simulink model "sensorFusionWithControlTB66State"  (R2024a)
settings: Solver=FixedStepAuto  StartTime=0.0  StopTime=inf  FixedStep=controlRate  RelTol=1e-3
InitFcn:
  | modelParamsDD = Simulink.data.dictionary.open('modelConfigData.sldd');
  | sectModel = getSection(modelParamsDD,'Design Data');
  | controlRateTemp = getValue(getEntry(sectModel,'controlRate'));
  | mpcRate = getValue(getEntry(sectModel,'mpcRate'));
  | 
  | measRate = controlRateTemp;
  | angleEstRate = measRate;
  | stateEstRate = measRate;
  | 
  | % Complementary filter
  | fc = 5; %Hz
  | tau = 1/(2*pi*fc);
  | % alpha = tau/(tau+controlRateTemp);
  | alpha = 0.98;
  | 
  | % Control params
  | tiltSetPoint = 5; % degree
  | 
  | % Motor params
  | % PPR = 13;
  | % gearReductionRatio = 42;
  | % ABPhase = 4;
  | 
  | % Tilt angle PID
  | Tw = 1;
  | Kp = 25;
  | Ki = 15; % At 100 Hz
  | Kd = 0;
  | 
  | clear controlRateTemp
  | 
  | motorParamsDD = Simulink.data.dictionary.open('motorParametersData.sldd');
  | robotParamsDD = Simulink.data.dictionary.open('robotModelData.sldd');
  | % controlParamsDD = Simulink.data.dictionary.open('controlVariablesData.sldd');
  | sectMotor = getSection(motorParamsDD,'Design Data');
  | sectRobot = getSection(robotParamsDD,'Design Data');
  | % sectControl = getSection(controlParamsDD,'Design Data');
  | 
  | % Physical Parameters
  | M = getValue(getEntry(sectRobot,'massOfCart'));    % mass of cart
  | m = getValue(getEntry(sectRobot,'massOfPendulum'));    % mass of pendulum
  | L = getValue(getEntry(sectRobot,'lengthToPendulumCenterOfMass'));    % length to pendulum center of mass
  | g = 9.81;   % gravity
  | I = getValue(getEntry(sectRobot,'inertiaOfPendulum'));  % inertia of pendulum
  | r = getValue(getEntry(sectRobot,'wheelRadius'));   % 5 cm wheel radius
  | 
  | % Servo motor state: i, omega
  | Rm = getValue(getEntry(sectMotor,'armatureResistance')); % motor resistance
  | Lm = getValue(getEntry(sectMotor,'armatureInductance')); % motor coil inductance
  | Km = getValue(getEntry(sectMotor,'motorTorqueConstantKm')); % motor torque constant
  | Kb = getValue(getEntry(sectMotor,'backEMFConstantKb')); % motor electrical consant
  | Kf = getValue(getEntry(sectMotor,'viscousFriction')); % viscous friction
  | J = getValue(getEntry(sectMotor,'motorInertia'));  % inertia of rotor
  | 
  | % Q_aug_lqr_temp = getValue(getEntry(sectControl,'Q_aug_lqr'));
  | % R_aug_lqr_temp = getValue(getEntry(sectControl,'R_aug_lqr'));
  | 
  | % States are x, dx/dt, phi, dphi/dt
  | % Outputs are x position and tilt angle
  | 
  | % Linearized state-space model of inverted pendulum
  | I_tot = m*L^2+I;
  | p = m^2*L^2 - I_tot*(M+m);
  | A_pend = [0 1 0 0;
  |           0 0 (m^2 * g * L^2)/p 0;
  |           0 0 0 1;
  |           0 0 -(M+m)/(m*L)*m^2*L^2*g/p 0];
  | 
  | B_pend = [0; -I_tot/p; 0; 1/(m*L)*(1+(M+m)*I_tot/p)];
  | 
  | C_pend = [1 0 0 0;
  |           0 0 1 0];
  | D_pend = zeros(2,1);
  | 
  | % Discretize System - for the augmented system
  | sysd = c2d(ss(A_pend, B_pend, C_pend, D_pend), measRate);
  | Ad_pend = single(sysd.A);
  | Bd_pend = single(sysd.B);
  | Cd_pend = single(sysd.C);
  | Dd_pend = single(sysd.D);
  | 
  | % State-space model: output is torque = Km * i
  | A_motor = [-Rm/L,   -Kb/Lm;
  |             Km/J, -Kf/J];
  | B_motor = [1/Lm;
  |            0];
  | C_motor = [Km*(1/r), 0];  % Output is torque = Km * i
  | D_motor = 0;
  | 
  | % Augment System: Force = torque / r
  | % States are x, dx/dt, phi, dphi/dt, i, w
  | % Outputs are x position and tilt angle
  | 
  | A_aug = [A_pend, B_pend*C_motor;
  |          zeros(2,4), A_motor];
  | 
  | B_aug = [B_pend*D_motor; B_motor];
  | 
  | C_aug = [C_pend, D_pend*C_motor];
  | n_aug = size(A_aug,1);
  | 
  | 
  | % Discretize System - for the augmented system
  | sysd = c2d(ss(A_aug, B_aug, C_aug, 0), measRate);
  | Ad_aug = single(sysd.A);
  | Bd_aug = single(sysd.B);
  | Cd_aug = single(sysd.C);
  | 
  | clear J Kt M m l g I r Q_lqr_temp R_lqr_temp dt
  | clear Rm Lm Km Kb Kf J
  | clear motorParamsDD robotParamsDD controlParamsDD modelParamsDD sectMotor sectRobot sectControl sectModel sysd
  | 
  | % LQR Controller matrices (moved here from SLDD to be tuned)
  | xm = 0.01;
  | xdm = 2;
  | pm = 0.2;
  | pdm = 5;
  | im = 2;
  | wm = 100;
  | 
  | Q_aug_lqr_temp = 0.1*diag([(1/xm)^2,(1/xdm)^2,(1/pm)^2,(1/pdm)^2,(1/im)^2,(1/wm)^2]);
  | R_aug_lqr_temp = 15;
  | 
  | % LQR Controller - for the augmented system
  | [K_aug_lqr, ~, ~] = dlqr(Ad_aug, Bd_aug, Q_aug_lqr_temp, R_aug_lqr_temp);
  | K_aug_lqr = single(K_aug_lqr);
  | 
  | clear Q_aug_lqr_temp R_aug_lqr_temp
  | 
  | %% MPC Tuning:
  | % Control Voltage was low, settling of the state variables is slow.
  | % Sol1: Decrease mpc1.Weights.MVRate (the penalty on voltage be cheaper)
  | % Sol2: Increase the weights penalty (same, more expensive error)
  | % Sol3: Initial conditions should not be near the constraints.
  | 
  | % For 1000 Hz sample rate with sensors, and 100 Hz sample rate MPC, the
  | % 200 long predict and 10 long control horizon should be enough,
  | % the system can't change faster.
  | 
  | % MPC tuning params
  | horizonNum = 100;
  | controlHorizon = 20;
  | 
  | MVWeight = 0;
  | MVRateWeight = 0.1;
  | stateVariableWeights = [0 0 1 0 0 0];
  | ECR = 100000;
  | 
  | % MPC Constraints
  | x_m = 2;
  | x_dot_m = 2;
  | phi_m = 1;
  | phi_dot_m = 35;
  | i_m = 10;
  | w_m = 200;
  | 
  | % MPC
  | robSys_mpc = c2d(ss(A_aug, B_aug, eye(6), zeros(6,1)), mpcRate);
  | %% create MPC controller object with sample time
  | mpc1 = mpc(robSys_mpc, mpcRate);
  | %% specify prediction horizon
  | mpc1.PredictionHorizon = horizonNum;
  | %% specify control horizon
  | mpc1.ControlHorizon = controlHorizon;
  | %% specify nominal values for inputs and outputs
  | mpc1.Model.Nominal.U = 0;
  | mpc1.Model.Nominal.Y = [0;0;0;0;0;0];
  | %% specify constraints for MV and MV Rate
  | mpc1.MV(1).Min = -12;
  | mpc1.MV(1).Max = 12;
  | %% specify constraints for OV
  | mpc1.OV(1).Min = -x_m;
  | mpc1.OV(1).Max = x_m;
  | mpc1.OV(2).Min = -x_dot_m;
  | mpc1.OV(2).Max = x_dot_m;
  | mpc1.OV(3).Min = -phi_m;
  | mpc1.OV(3).Max = phi_m;
  | mpc1.OV(4).Min = -phi_dot_m;
  | mpc1.OV(4).Max = phi_dot_m;
  | mpc1.OV(5).Min = -i_m;
  | mpc1.OV(5).Max = i_m;
  | mpc1.OV(6).Min = -w_m;
  | mpc1.OV(6).Max = w_m;
  | %% specify weights
  | mpc1.Weights.MV = MVWeight;
  | mpc1.Weights.MVRate = MVRateWeight;
  | mpc1.Weights.OV = stateVariableWeights;
  | mpc1.Weights.ECR = ECR;
  | %% specify overall adjustment factor applied to estimation model gains
  | alphaMPC = 4.1687;
  | %% adjust default output disturbance model gains
  | setoutdist(mpc1, 'model', getoutdist(mpc1)*0);
  | %% adjust default measurement noise model gains
  | mpc1.Model.Noise = mpc1.Model.Noise*0;
  | %% specify simulation options
  | options = mpcsimopt();
  | options.RefLookAhead = 'off';
  | options.MDLookAhead = 'off';
  | options.Constraints = 'on';
  | options.OpenLoop = 'off';
  | 
  | setEstimator(mpc1,'custom')
undefined symbols (not defined in the file or in its folder): accelToUnit, controlRate, gyroToUnit, MaxMotorVoltage
libraries: stm32blockslib x2, stm32f7xxblockslib x2, stm32f4xxblockslib x1
settings Model: DataDictionary=globalData.sldd  VariantConfigurationObject=RobotVariantConfig  STM32="{\"PWMOutput\":[{\"ID\":\"sensorFusionWithControlTB66State:205\"},{\"ID\":\"sensorFusionWithControlTB66State:189\"}],\"DigitalPortWrite\":[{\"ID\":\"sensorFusionWithControlTB66State:1189\"},{\"ID\":\"sensorFusionWithControlTB66State:1225:7\"},{\"ID\":\"sensorFusionWithControlTB66State:1225:8\"},{\"ID\":\"sensorFusionWithControlTB66State:1225:9\"},{\"ID\":\"sensorFusionWithControlTB66State:1225:10\"}],\"EncoderBlock\":[{\"ID\":\"sensorFusionWithControlTB66State:1254\"},{\"ID\":\"sensorFusionWithControlTB66State:1257\"}],\"I2CControllerRead\":[{\"ID\":\"sensorFusionWithControlTB66State:1237:7\"},{\"ID\":\"sensorFusionWithControlTB66State:1237:18\"},{\"ID\":\"sensorFusionWithControlTB66State:1237:19\"},{\"ID\":\"sensorFusionWithControlTB66State:1237:20\"},{\"ID\":\"sensorFusionWithControlTB66State:1238:7\"},{\"ID\":\"sensorFusionWithControlTB66State:1238:15\"},{\"ID\":\"sensorFusionWithControlTB66State:1238:16\"},{\"ID\":\"sensorFusionWithControlTB66State:1238:17\"}],\"I2CControllerWrite\":[{\"ID\":\"sensorFusionWithControlTB66State:1237:21\"},{\"ID\":\"sensorFusionWithControlTB66State:1237:22\"},{\"ID\":\"sensorFusionWithControlTB66State:1237:23\"},{\"ID\":\"sensorFusionWithControlTB66State:1238:18\"},{\"ID\":\"sensorFusionWithControlTB66State:1238:19\"},{\"ID\":\"sensorFusionWithControlTB66State:1238:20\"}]}"  SimulationMode=external  Creator=Peter  LastModifiedBy=Peter
settings SolverCC: PositivePriorityOrder=on
settings OptimizationCC: OptimizeBlockIOStorage=off  BufferReuse=off  ReuseModelBlockBuffer=off  GlobalBufferReuse=off  ExpressionFolding=off  EnableMemcpy=off  PassReuseOutputArgsAs=Individual arguments  LocalBlockOutputs=off  ZeroExternalMemoryAtStartup=off  ZeroInternalMemoryAtStartup=off  MaxStackSize=64  OptimizeDataStoreBuffers=off  BusAssignmentInplaceUpdate=off  OptimizationLevel=level0  OptimizationCustomize=off  EfficientTunableParamExpr=on
settings DebuggingCC: ParameterTunabilityLossMsg=error
settings HardwareCC: ProdBitPerPointer=32  ProdBitPerSizeT=32  ProdBitPerPtrDiffT=32  ProdLargestAtomicInteger=Long  ProdLargestAtomicFloat=Double  ProdWordSize=32  ProdLongLongMode=on  ProdHWDeviceType=ARM Compatible->ARM Cortex-M
settings SFSimCC: MATLABDynamicMemAlloc=off
settings RTWCC: Description=Embedded Coder  SystemTargetFile=ert.tlc  HardwareBoard=STM32F7xx Based (Single precision FPU)  TemplateMakefile=ert_default_tmf  Toolchain=GNU Tools for ARM Embedded Processors
settings CodeAppCC: GenerateComments=off  IgnoreCustomStorageClasses=off  OperatorAnnotations=on  SimulinkDataObjDesc=on  SFDataObjDesc=on  SimulinkBlockComments=off
settings ERTTargetCC: TargetLangStandard=C99 (ISO)  CodeReplacementLibrary=ARM Cortex-M  SupportComplex=off  ExtMode=on  ExtModeTransport=3  ExtModeStaticAlloc=on  ExtModeStaticAllocSize=2048  ExtModeMexFile=ext_xcp  ExtModeMexArgs=1 'COM11' 115200  ExtModeIntrfLevel=Level2 - Open

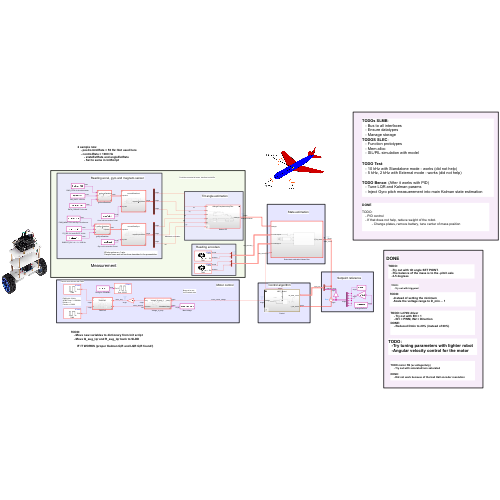
[thumbnail: Simulink's stored preview of the top-level diagram]
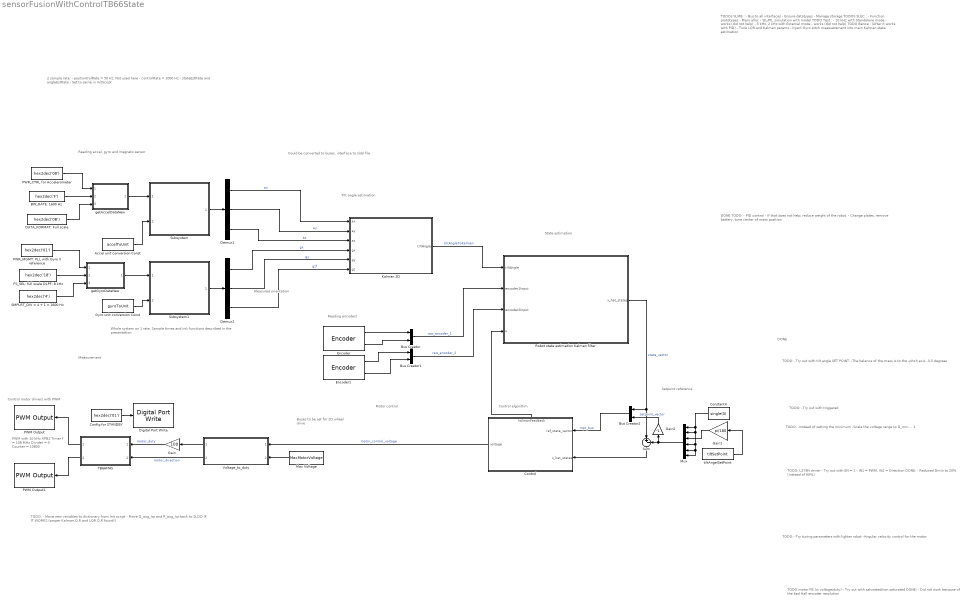
== system sensorFusionWithControlTB66State ==
  note: 2 sample rate:
      | - posControlRate = 50 Hz: Not used here
      | - controlRate = 1000 Hz
      | - stateEstRate and angleEstRate
      | - Set to same in InitScript
  note: Measured orientation
  note: PWM with 10 kHz
      | APB2 Timer f = 108 MHz
      | Divider = 0
      | Counter = 10800
  note: Measurement
  note: Motor control
  note: Tilt angle estimation
  note: Control motor dirvers with PWM
  note: Reading accel, gyro and megneto sensor
  note: Control algorithm
  note: Reading encoders
  note: State estimation
  note: Setpoint reference
  note: Could be converted to buses, interface to sldd file
  note: Whole system on 1 rate.
      | Sample times and init functions described in the presentation.
  note: Buses to be set
      | for 2D wheel drive
  note: TODO:
      | -Try tuning parameters with lighter robot
      | -Angular velocity control for the motor
  note: TODO motor FB (w voltage/duty)
      | - Try out with saturated/non saturated
      |
      | DONE:
      | - Did not work because of the bad Hall encoder resolution
  note: TODO:
      | -Try out with tilt angle SET POINT.
      | -The balance of the mass is to the -pitch axis
      | -3-5 degrees
  note: TODO: L279N driver
      | - Try out with EN = 1
      | - IN1 = PWM, IN2 = Direction
      | DONE:
      | - Reduced Dmin to 20% (instead of 60%)
  note: TODOs SLMB :
      | - Bus to all interfaces
      | - Ensure datatypes
      | - Manage storage
      | TODOS SLEC :
      | - Function prototypes
      | - Mem alloc
      | - SIL/PIL simulation with model
      |
      | TODO Test :
      | - 10 kHz with Standalone mode - works (did not help)
      | - 5 kHz, 2 kHz with External mode - works (did not help)
      |
      | TODO Bence : (After it works with PID)
      | - Tune LQR and Kalman params
      | - Inject Gyro pitch measuerement into main Kalman state estimation
  note: TODO:
      | -Try out with triggered
  note: DONE
  note: DONE
      |
      | TODO:
      | - PID control
      | - If that does not help, reduce weight of the robot.
      | - Change plates, remove battery, tune center of mass position
  note: TODO:
      | -Instead of setting the minimum
      | -Scale the voltage range to D_min ... 1
  note: TODO:
      | - Move new variables to dictionary from Init script
      | - Move Q_aug_lqr and R_aug_lqr back to SLDD
      |
      | IF IT WORKS (proper Kalman Q,R and LQR Q,R found!)
  Accel unit conversion Const : Constant  Value=accelToUnit  OutDataTypeStr=single
  BW_RATE: 1600 Hz : Constant  Value=hex2dec('F')  OutDataTypeStr=uint8
  Bus Creator : BusCreator  Inputs=2
  Bus Creator1 : BusCreator  Inputs=2
  Bus Creator2 : BusCreator  Inputs=2
  Config for STANDBY : Constant  Value=hex2dec('01')  OutDataTypeStr=uint8
  Constant4 : Constant  Value=single(0)
  Control : Subsystem  Variant=on  VariantChoicesEnumeration=controlEnumState  VariantControlVariable=controlAlgStateCtrl  VariantControl=Subsystem2  VariantActivationTime=inherit from Simulink.VariantControl
      settings: PortSchema="{\"entries\":[{\"content\":{\"sides\":[{\"content\":{\"connectorIds\":[\"In1\",\"In2\"]},\"type\":\"ConnectorPlacement.EquallySpacedRectSide\",\"uuid\":\"f699f757-4844-4aff-9ceb-41d5b2044f89\"},{\"content\":{\"connectorIds\":[\"Out1\"],\"side\":\"RIGHT\"},\"type\":\"ConnectorPlacement.EquallySpacedRectSide\",\"uuid\":\"5d4ff76b-5e14-4a3a-b7d6-9f05c394657c\"},{\"content\":{\"connectorIds\":[\"Out2\"],\"side\":\"TOP\"},\"type\":\"ConnectorPlacement.EquallySpacedRectSide\",\"uuid\":\"774b8687-b42a-4b88-b210-7c8eb4b61568\"}]},\"type\":\"ConnectorPlacement.EquallySpacedConnector\",\"uuid\":\"f6913896-c1bf-44b7-bb24-894f4bed7d15\"}],\"packageUris\":[\"http://schema.mathworks.com/mf0/Connector/R2020b\"],\"version\":\"1.0\"}"
  DATA_FORMAT: Full scale : Constant  Value=hex2dec('0B')  OutDataTypeStr=uint8
  Demux1 : Demux  Outputs=3
  Demux2 : Demux  Outputs=3
  Digital Port Write : stm32f4xxblockslib/Digital Port Write  PortName=GPIOF  PinNumber=[13]  ReadOperation=off  IOAsArray=off  EnableSimPort=off  hoistedMaskSrc=ECSoC/ECSimCodegen/Digital Port Write
      settings: LibrarySourceBlock=stm32f7xxblockslib/Digital Port Write
  Encoder : stm32blockslib/Encoder  TimerModule=TIM1  EnableResetInput=off  OutputDirection=on  SampleTime=angleEstRate
      settings: LibrarySourceBlock=stm32f7xxblockslib/Encoder
  Encoder1 : stm32blockslib/Encoder  TimerModule=TIM3  EnableResetInput=off  OutputDirection=on  SampleTime=angleEstRate
      settings: LibrarySourceBlock=stm32f7xxblockslib/Encoder
  FS_SEL: full scale DLPF: 8 kHz : Constant  Value=hex2dec('18')  OutDataTypeStr=uint8
  Gain : Gain  Gain=100
  Gain1 : Gain  Gain=pi/180  ParamDataTypeStr=single
  Gain2 : Gain  Gain=-1
  Gyro unit conversion Const : Constant  Value=gyroToUnit  OutDataTypeStr=single
  Kalman 2D : Subsystem  Variant=on  VariantChoicesEnumeration=tiltEnum  VariantControlVariable=tiltEstCtrl  VariantControl=Kalman 2D  VariantActivationTime=inherit from Simulink.VariantControl
  Max Voltage : Constant  Value=MaxMotorVoltage  OutDataTypeStr=single
  Mux : Mux  Inputs=6
  PWM Output : stm32f7xxblockslib/PWM Output  TimerModule=TIM8  DutycycleUnits=Percentage  EnableChannel1=off  EnableChannel2=off  EnableChannel3=on  EnableChannel4=off  EnableChannel5=off  EnableChannel6=off  EnableCounterInput=off  EnableMainOutputInput=off  EnableFrequencyInput=off  SetRCAfterCE=off  OutputDirection=off  OutputMainOutputEnableStatus=off  SampleTime=0.1  EnableSimPort=off  EnableUpdateEvent=off  EnableCaptureCompare1Event=off  EnableCaptureCompare2Event=off  EnableCaptureCompare3Event=off  EnableCaptureCompare4Event=off  EnableTriggerEvent=off  EnableBreakEvent=off  EnableBreakEvent2=off  ProcessorFamily=STM32F7  hoistedMaskSrc=ECSoC/ECSimCodegen/PWM Output
  PWM Output1 : stm32f7xxblockslib/PWM Output  TimerModule=TIM8  DutycycleUnits=Percentage  EnableChannel1=off  EnableChannel2=off  EnableChannel3=off  EnableChannel4=on  EnableChannel5=off  EnableChannel6=off  EnableCounterInput=off  EnableMainOutputInput=off  EnableFrequencyInput=off  SetRCAfterCE=off  OutputDirection=off  OutputMainOutputEnableStatus=off  SampleTime=0.1  EnableSimPort=off  EnableUpdateEvent=off  EnableCaptureCompare1Event=off  EnableCaptureCompare2Event=off  EnableCaptureCompare3Event=off  EnableCaptureCompare4Event=off  EnableTriggerEvent=off  EnableBreakEvent=off  EnableBreakEvent2=off  ProcessorFamily=STM32F7  hoistedMaskSrc=ECSoC/ECSimCodegen/PWM Output
  PWR_CTRL for Accelerometer : Constant  Value=hex2dec('08')  OutDataTypeStr=uint8
  PWR_MGMT: PLL with Gyro X reference : Constant  Value=hex2dec('01')  OutDataTypeStr=uint8
  Robot state estimation Kalman filter : Subsystem  TreatAsAtomicUnit=on  SystemSampleTime=stateEstRate
  SMPLRT_DIV = 4 + 1 = 1600 Hz : Constant  Value=hex2dec('4')  OutDataTypeStr=uint8
  Subsystem : Subsystem  TreatAsAtomicUnit=on  SystemSampleTime=angleEstRate  ReferencedSubsystem=convertRawAccel
  Subsystem1 : Subsystem  TreatAsAtomicUnit=on  SystemSampleTime=angleEstRate  ReferencedSubsystem=convertRawGyro
  Sum : Sum  Inputs=|+-
  TB66FNG : Subsystem  TreatAsAtomicUnit=on  SystemSampleTime=controlRate  ReferencedSubsystem=TB66FNG
  Voltage_to_duty : Subsystem  TreatAsAtomicUnit=on  SystemSampleTime=controlRate  ReferencedSubsystem=Voltage_to_duty_1
  getAccelDataNew : Subsystem  TreatAsAtomicUnit=on  ReferencedSubsystem=getAccelDataNew
  getGyroDataNew : Subsystem  TreatAsAtomicUnit=on  ReferencedSubsystem=getGyroDataNew
  tiltAngelSetPoint : Constant  Value=tiltSetPoint  OutDataTypeStr=single
  wires:
  Max Voltage/1 -> Voltage_to_duty/2
  Gyro unit conversion Const/1 -> Subsystem1/2
  Subsystem1/1 -> Demux2/1
  PWR_MGMT: PLL with Gyro X reference/1 -> getGyroDataNew/1
  getGyroDataNew/1 -> Subsystem1/1
  Kalman 2D/1(tiltAngle) -> Robot state estimation Kalman filter/1(tiltAngle)  "tiltAngleToKalman"
  Demux1/1 -> Kalman 2D/1(ax)  "ax"
  Demux1/2 -> Kalman 2D/2(ay)  "ay"
  Demux1/3 -> Kalman 2D/3(az)  "az"
  Demux2/3 -> Kalman 2D/6(gz)  "gzf"
  getAccelDataNew/1 -> Subsystem/1
  Accel unit conversion Const/1 -> Subsystem/2
  Subsystem/1 -> Demux1/1
  Control/1(voltage) -> Voltage_to_duty/1  "motor_control_voltage"
  Demux2/1 -> Kalman 2D/4(gx)  "gx"
  Demux2/2 -> Kalman 2D/5(gy)  "gy"
  BW_RATE: 1600 Hz/1 -> getAccelDataNew/2
  PWR_CTRL for Accelerometer/1 -> getAccelDataNew/1
  FS_SEL: full scale DLPF: 8 kHz/1 -> getGyroDataNew/2
  SMPLRT_DIV = 4 + 1 = 1600 Hz/1 -> getGyroDataNew/3
  Sum/1 -> Control/2(x_hat_states)
  Mux/1 -> Gain2/1, Sum/2
  Constant4/1 -> Mux/6, Mux/5, Mux/4, Mux/2, Mux/1
  tiltAngelSetPoint/1 -> Gain1/1
  Voltage_to_duty/1 -> Gain/1
  Voltage_to_duty/2 -> TB66FNG/2  "motor_direction"
  TB66FNG/1 -> PWM Output/1
  TB66FNG/2 -> PWM Output1/1
  Config for STANDBY/1 -> Digital Port Write/1
  DATA_FORMAT: Full scale/1 -> getAccelDataNew/3
  Gain1/1 -> Mux/3
  Encoder/1 -> Bus Creator/1
  Encoder1/1 -> Bus Creator1/1
  Bus Creator/1 -> Robot state estimation Kalman filter/2(encoder1Input)  "raw_encoder_1"
  Encoder/2 -> Bus Creator/2
  Encoder1/2 -> Bus Creator1/2
  Bus Creator1/1 -> Robot state estimation Kalman filter/3(encoder2Input)  "raw_encoder_2"
  Robot state estimation Kalman filter/1(x_hat_states) -> Sum/1, Bus Creator2/1  "state_vector"
  Gain/1 -> TB66FNG/1  "motor_duty"
  Bus Creator2/1 -> Control/1(ref_state_vector)  "mpc_bus"
  Control/2(kalmanFeedback) -> Robot state estimation Kalman filter/4(u)
  Gain2/1 -> Bus Creator2/2  "setpoint_vector"

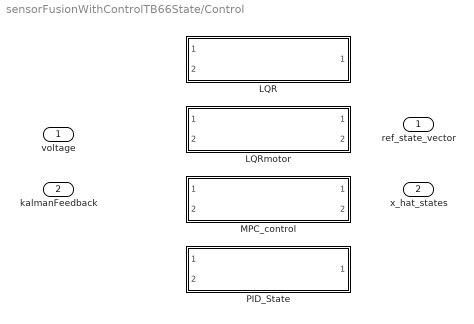
== system sensorFusionWithControlTB66State/Control ==
  ref_state_vector : Inport
  x_hat_states : Inport  Port=2  OutDataTypeStr=single
  LQR : Subsystem  SystemSampleTime=controlRate  VariantControl=controlAlgStateCtrl == controlEnumState.LQR  ReferencedSubsystem=LQR
  LQRmotor : Subsystem  SystemSampleTime=controlRate  VariantControl=controlAlgStateCtrl == controlEnumState.LQRmotor  ReferencedSubsystem=LQRmotor
  MPC_control : Subsystem  VariantControl=controlAlgStateCtrl == controlEnumState.MPC_control  ReferencedSubsystem=MPC_control
  PID_State : Subsystem  VariantControl=controlAlgStateCtrl == controlEnumState.PID_State  ReferencedSubsystem=PID_State
  voltage : Outport  OutDataTypeStr=single
  kalmanFeedback : Outport  Port=2  OutDataTypeStr=single

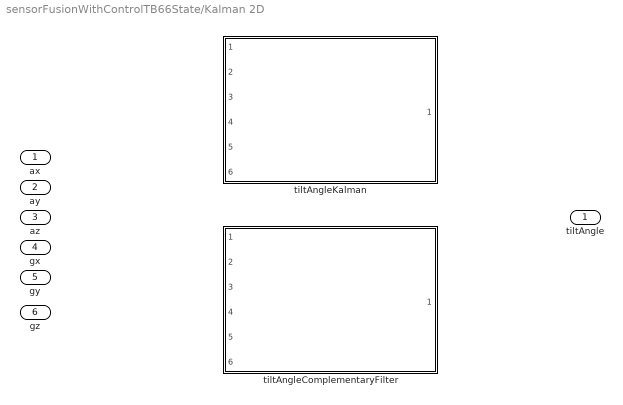
== system sensorFusionWithControlTB66State/Kalman 2D ==
  ax : Inport
  ay : Inport  Port=2
  az : Inport  Port=3
  gx : Inport  Port=4
  gy : Inport  Port=5
  gz : Inport  Port=6
  tiltAngleComplementaryFilter : Subsystem  TreatAsAtomicUnit=on  SystemSampleTime=controlRate  VariantControl=tiltEstCtrl == tiltEnum.tiltAngleComplementaryFilter  ReferencedSubsystem=tiltAngleComplementaryFilter
  tiltAngleKalman : Subsystem  TreatAsAtomicUnit=on  SystemSampleTime=angleEstRate  VariantControl=tiltEstCtrl == tiltEnum.tiltAngleKalman  ReferencedSubsystem=tiltAngleKalman
  tiltAngle : Outport

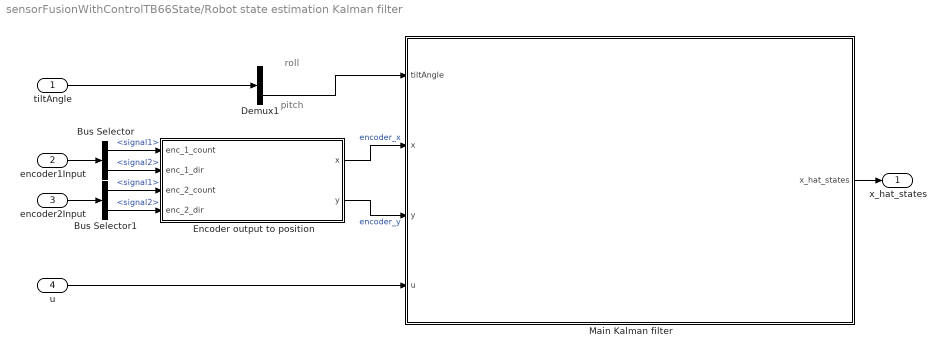
== system sensorFusionWithControlTB66State/Robot state estimation Kalman filter ==
  note: pitch
  note: roll
  tiltAngle : Inport
  encoder1Input : Inport  Port=2
  encoder2Input : Inport  Port=3
  u : Inport  Port=4
  Bus Selector : BusSelector  OutputSignals=signal1,signal2
  Bus Selector1 : BusSelector  OutputSignals=signal1,signal2
  Demux1 : Demux  Outputs=2
  Encoder output to position : Subsystem  Variant=on  VariantChoicesEnumeration=encoderDimEnum  VariantControlVariable=encoderDimCtrl  VariantControl=Encoder output to position  VariantActivationTime=inherit from Simulink.VariantControl
  Main Kalman filter : Subsystem  Variant=on  VariantChoicesEnumeration=mainStateEnum  VariantControlVariable=mainStateEstCtrl  VariantControl=Subsystem1  VariantActivationTime=inherit from Simulink.VariantControl
  x_hat_states : Outport  OutDataTypeStr=single
  wires:
  tiltAngle/1 -> Demux1/1
  Main Kalman filter/1(x_hat_states) -> x_hat_states/1
  Bus Selector/1 -> Encoder output to position/1(enc_1_count)  "<signal1>"
  Bus Selector/2 -> Encoder output to position/2(enc_1_dir)  "<signal2>"
  Encoder output to position/1(x) -> Main Kalman filter/2(x)  "encoder_x"
  Encoder output to position/2(y) -> Main Kalman filter/3(y)  "encoder_y"
  u/1 -> Main Kalman filter/4(u)
  Demux1/2 -> Main Kalman filter/1(tiltAngle)
  encoder1Input/1 -> Bus Selector/1
  encoder2Input/1 -> Bus Selector1/1
  Bus Selector1/1 -> Encoder output to position/3(enc_2_count)  "<signal1>"
  Bus Selector1/2 -> Encoder output to position/4(enc_2_dir)  "<signal2>"

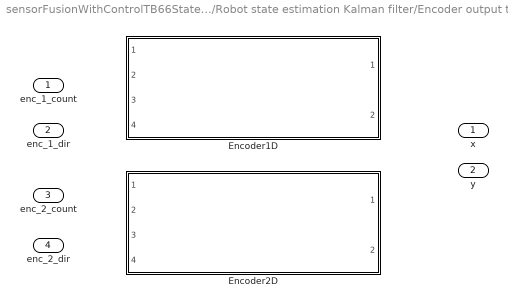
== system sensorFusionWithControlTB66State/Robot state estimation Kalman filter/Encoder output to position ==
  enc_1_count : Inport
  enc_1_dir : Inport  Port=2
  enc_2_count : Inport  Port=3
  enc_2_dir : Inport  Port=4
  Encoder1D : Subsystem  VariantControl=encoderDimCtrl == encoderDimEnum.Encoder1D  ReferencedSubsystem=Encoder1D
  Encoder2D : Subsystem  VariantControl=encoderDimCtrl == encoderDimEnum.Encoder2D  ReferencedSubsystem=Encoder2D
  x : Outport  OutDataTypeStr=single
  y : Outport  Port=2  OutDataTypeStr=single

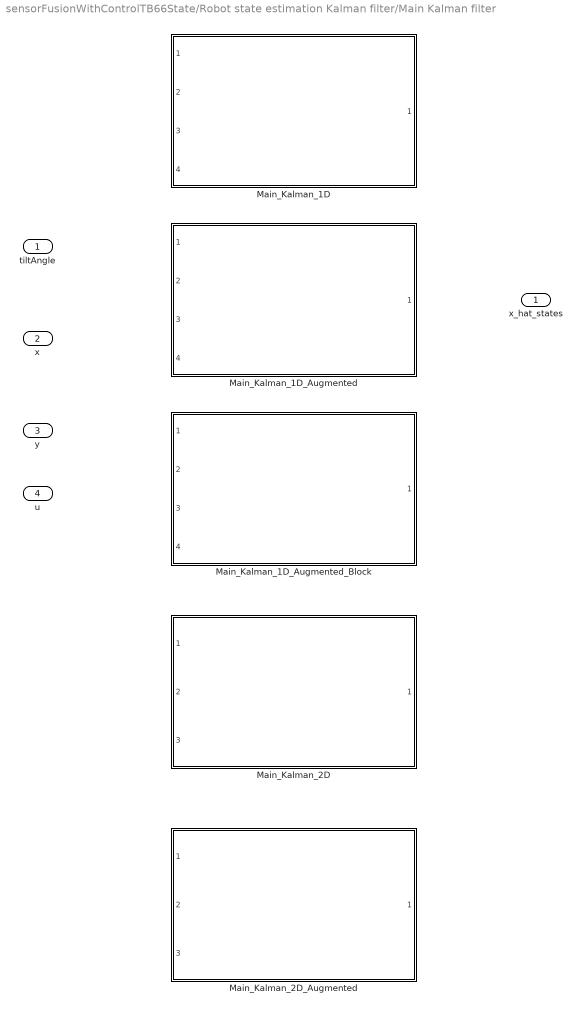
== system sensorFusionWithControlTB66State/Robot state estimation Kalman filter/Main Kalman filter ==
  tiltAngle : Inport  OutDataTypeStr=single
  x : Inport  Port=2  OutDataTypeStr=single
  y : Inport  Port=3  OutDataTypeStr=single
  u : Inport  Port=4  OutDataTypeStr=single
  Main_Kalman_1D : Subsystem  VariantControl=mainStateEstCtrl == mainStateEnum.Main_Kalman_1D  ReferencedSubsystem=Main_Kalman_1D
  Main_Kalman_1D_Augmented : Subsystem  VariantControl=mainStateEstCtrl == mainStateEnum.Main_Kalman_1D_Augmented  ReferencedSubsystem=Main_Kalman_1D_Augmented
  Main_Kalman_1D_Augmented_Block : Subsystem  VariantControl=mainStateEstCtrl == mainStateEnum.Main_Kalman_1D_Augmented_Block  ReferencedSubsystem=Main_Kalman_1D_Augmented_Block
  Main_Kalman_2D : Subsystem  VariantControl=mainStateEstCtrl == mainStateEnum.Main_Kalman_2D  ReferencedSubsystem=Main_Kalman_2D
  Main_Kalman_2D_Augmented : Subsystem  VariantControl=mainStateEstCtrl == mainStateEnum.Main_Kalman_2D_Augmented  ReferencedSubsystem=Main_Kalman_2D_Augmented
  x_hat_states : Outport  OutDataTypeStr=single
